simulink model "Equ7_2_2"  (Simulink 8.9)
settings: Solver=ode45  StartTime=0.0  StopTime=20  RelTol=1e-3  EnableMultiTasking=on
undefined symbols (not defined in the file): I, K, Kd
libraries: dspsrcs4 x1
settings Model: SuppressorTable=22 serialization::archive 11 0 6 0 0 0 0 0  Creator=Anita Enmark  LastModifiedBy=pechorin
settings OptimizationCC: ExpressionDepthLimit=2147483647  InitFltsAndDblsToZero=on
settings DebuggingCC: SaveWithParameterizedLinksMsg=none  SignalResolutionControl=TryResolveAllWithWarning  SolverPrmCheckMsg=warning
settings GRTTargetCC: TargetFcnLib=ansi_tfl_tmw.mat

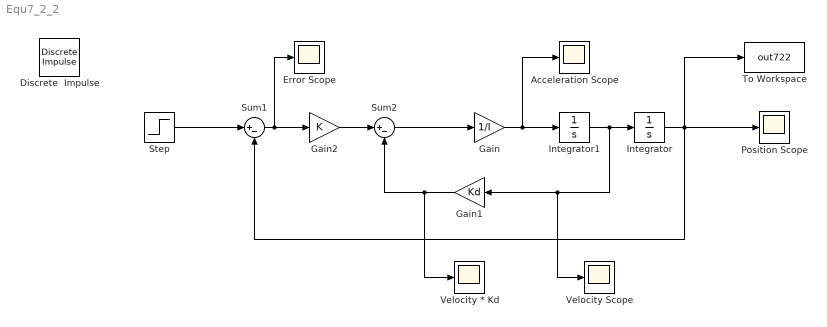
== system Equ7_2_2 ==
  Acceleration Scope : Scope
  Discrete  Impulse : dspsrcs4/Discrete  Impulse  Delay=0  SampleTime=1  FrameSample=1  OutputFrames=off  dataType=double  isSigned=on  wordLen=16  udDataType=sfix(16)  fracBitsMode=Best precision  numFracBits=15  OutDataTypeStr=double  LastOutDataTypeStr=double
  Error Scope : Scope
  Gain : Gain  Gain=1/I
  Gain1 : Gain  Gain=Kd
  Gain2 : Gain  Gain=K
  Integrator : Integrator
  Integrator1 : Integrator
  Position Scope : Scope
  Step : Step  Time=0  SampleTime=0
  Sum1 : Sum  Inputs=|+-
  Sum2 : Sum  Inputs=|+-
  To Workspace : ToWorkspace  VariableName=out722  SaveFormat=Timeseries  SampleTime=-1
  Velocity * Kd : Scope
  Velocity Scope : Scope
  wires:
  Integrator1/1 -> Integrator/1, Velocity Scope/1, Gain1/1
  Integrator/1 -> Position Scope/1, Sum1/2, To Workspace/1
  Gain/1 -> Acceleration Scope/1, Integrator1/1
  Sum1/1 -> Gain2/1, Error Scope/1
  Gain1/1 -> Sum2/2, Velocity * Kd/1
  Sum2/1 -> Gain/1
  Gain2/1 -> Sum2/1
  Step/1 -> Sum1/1
